simulink library "EmE_MBD_Blockset"  (R2018a)
settings: Solver=ode1  StartTime=0.0  StopTime=Inf  FixedStep=0.001  RelTol=1e-3  EnableMultiTasking=on
PostLoadFcn:
  | , if any(exist('dsrtsu_mdlpostloadfcn', 'file') == [2, 3, 6]), try dsrtsu_mdlpostloadfcn('Execute', bdroot); catch fprintf('Error in PostLoadFcn (dsrtsu_mdlpostloadfcn) for model "%s":\n %s\n', bdroot, lasterr); end, end,
undefined symbols (not defined in the file or in its folder): ENUM_TSC1_CONTROL_PURPOSE_T, gcbh, GLB_SWITCH_T
libraries: simulink x237, $bdroot x115, simulink_need_slupdate x26, MotoHawk_lib x13, simulink_extras x3
(part 1 of 11)
settings Model: DSRTSU_INTERNAL_RTI_VER=520  DSRTSU_INTERNAL_RTI_TYPE=rti1401  DSRTSU_INTERNAL_RTIFPGA=110  RTICANMMDATA=struct('GeneralSetupData',struct('modelroot','C:\data\svn\PowerTrainSys\trunk\src\Projects_RCP\MY2017_RCP\EmE_MBD_Blockset','generalsettings',struct('filesettings',struct('destfolder',struct('Name','RTICANMM_FILES','Check',1),'buildfolder',struct('Name','.','Check',1),'AbsDestfolder',struct('Name','C:\data\svn\PowerTrainSys\trunk\src\Projects_RCP\MY2017_RCP\EmE_MBD_Blockset\RTICANMM_FILES'),'AbsBuildfolder',struct('Name','C:\data\svn\PowerTrainSys\trunk\src\Projects_RCP\MY2017_RCP\EmE_MBD_Blockset'))),'options',struct('addpaths',1,'rmpaths',1,'addtrcexclusion',logical(1),'cannavigator',struct('checkmonitoring',0),'show_usrtrc',0,'use_usrtrc',0),'advanced',struct('options',[1 1 1 1 1 1 1 1 1 1 1 1 1 1 1 1 1 1 1 1 1 1 1 1 1 1 1 1 1 1 1 1 1 1 1 1 1 1 1 1 1 1 1 1 1 1 1 1 1 1 1 1 1 1 1 1 1 1 1 1 1 1 1 1 1 1 1 1 1 1 1 1 1 1 1 1 1 1 1 1 1 1 1 1 1 1 1 1 1 1 1 1 1 1 1 1 1 1 1 1]),'MPSetup',{{}},'modelname','EmE_MBD_Blockset','block','EmE_MBD_Blockset'))  DSRTSU_INTERNAL_RTIFLEXRAYCONFIG=110  Creator=Charles.Swart  LastModifiedBy=Charles.Swart
settings DataIOCC: LimitDataPoints=on  SaveFormat=Array
settings OptimizationCC: BlockReduction=off  OptimizeBlockIOStorage=off  BufferReuse=off  GlobalBufferReuse=off  ExpressionFolding=off  LocalBlockOutputs=off  LifeSpan=inf  OptimizeDataStoreBuffers=off  BusAssignmentInplaceUpdate=off
settings DebuggingCC: SolverPrmCheckMsg=warning  SFUnexpectedBacktrackingDiag=warning  SFNoUnconditionalDefaultTransitionDiag=warning  SFExecutionAtInitializationDiag=none
settings HardwareCC: ProdBitPerPointer=32  ProdBitPerSizeT=32  ProdBitPerPtrDiffT=32  ProdLargestAtomicInteger=Integer  ProdEndianess=BigEndian  ProdWordSize=32  ProdHWDeviceType=Generic->Custom  TargetIntDivRoundTo=Zero  TargetEndianess=BigEndian  TargetHWDeviceType=Generic->Custom
settings ModelReferenceCC: PropagateSignalLabelsOutOfModel=off
settings SFSimCC: MATLABDynamicMemAlloc=off
settings RTWCC: SystemTargetFile=rti1401.tlc  MakeCommand=make_rti  TemplateMakefile=rti1401.tmf  Description=dSPACE DS1401 Hardware Platform
settings CodeAppCC: StateflowObjectComments=on
settings STFCustomTargetCC: ParMdlRefBuildCompliant=on  GeneratePreprocessorConditionals=Disable all  MatFileLogging=on  GRTInterface=off  SystemTargetFile=rti1401.tlc
settings GRTTargetCC: TargetLangStandard=C89/C90 (ANSI)  CompOptLevelCompliant=off  ConcurrentExecutionCompliant=off  GeneratePreprocessorConditionals=Disable all  CombineOutputUpdateFcns=off  CPPClassGenCompliant=off  UseToolchainInfoCompliant=off  ExtModeMexFile=noextcomm
settings ConfigComp: CovMetricSettings=dw  CovHtmlReporting=on  CovSaveCumulativeToWorkspaceVar=on  CovSaveSingleToWorkspaceVar=on  CovExternalEMLEnable=off  CovSFcnEnable=off

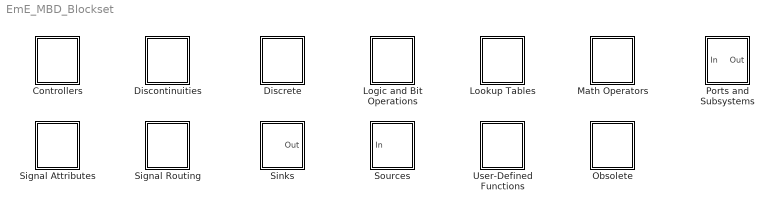
== system EmE_MBD_Blockset ==
  Controllers : Subsystem  mask(Define discontinuous states){}
      mask Display: image(imread('control.bmp','bmp'))
  Discontinuities : Subsystem  mask(Define discontinuous states){}
      mask Display: image(imread('nonlinear.bmp','bmp'))
  Discrete : Subsystem  mask(Define discrete states){}
      mask Display: image(imread('discrete.bmp','bmp'))
  Logic and Bit Operations : Subsystem  mask(Perform logic and bit operations){}
      mask Display: image(imread('logical_bit.bmp','bmp'))
  Lookup Tables : Subsystem  mask(Support lookup tables){}
      mask Display: image(imread('functions.bmp','bmp'))
  Math Operators : Subsystem  mask(Perform math operations){}
      mask Display: image(imread('math.bmp','bmp'))
  Obsolete : Subsystem  mask(Obsolete functions){}
      mask Display:
      | color('gray')
      | disp('X X X')
  Ports and Subsystems : Subsystem  mask(Support ports and subsystems){}
      mask Display: image(imread('subsystems.bmp','bmp'))
  Signal Attributes : Subsystem  mask(Support signal attributes){}
      mask Display: image(imread('attributes.bmp','bmp'))
  Signal Routing : Subsystem  mask(Support signal routing){}
      mask Display: image(imread('signals.bmp','bmp'))
  Sinks : Subsystem  mask(Receive output from other blocks){}
      mask Display: image(imread('sinks.bmp','bmp'))
  Sources : Subsystem  mask(Input to other blocks){}
      mask Display: image(imread('sources.bmp','bmp'))
  User-Defined Functions : Subsystem  mask(User-defined functions){}
      mask Display: image(imread('functions.bmp','bmp'))

== system EmE_MBD_Blockset/Controllers ==
  Generic_PID_Governor_3 : Subsystem  mask(Generic PID governor v3){}
      mask help:
      | Generic feedback governor v3 with proportional, integral, and derivative action (PID).
      | Anti-windup is achieved with a specified hysteresis limit value and a toggleable output unlimited vs. output limited delta feedback.
      | Derivative action has a optional configurable parameter to operate at specified multiples of the dT.
      | If GPID_slew_init is connected to GPID_setpoint, then the GPID_control_error value will be =(GPID_setpoint-GPID_feedback) upon a reset.
      | If GPID_slew_init is connected to GPID_feedback, then the GPID_control_error value will be =0 upon a reset.
      |
      | Do NOT connect GPID_slew_init to the GPID_setpoint port if using negative gains; else the integrator will initialize with a large negative value.
  Generic_PID_Governor_4 : Subsystem  mask(Generic PID governor 4 (EmE)){}
      mask help:
      | Generic feedback governor v4 with proportional, integral, and derivative action (PID).
      | Anti-windup is achieved with a specified hysteresis limit value and a toggleable output unlimited vs. output limited delta feedback.
      | Derivative action has a optional configurable parameter to operate at specified multiples of the dT.
      | If GPID_slew_init is connected to GPID_setpoint, then the GPID_control_error value will be =(GPID_setpoint-GPID_feedback) upon a reset.
      | If GPID_slew_init is connected to GPID_feedback, then the GPID_control_error value will be =0 upon a reset.
      |
      | Do NOT connect GPID_slew_init to the GPID_setpoint port if using negative gains; else the integrator will initialize with a large negative value.
      mask Display: % GPID_AW_USE_FEEDBACK_DELTA_CPV
  PID_saturating_terms : Subsystem  mask(PID governor (EmE)){}
      mask help:
      | PID governor with proportional, integral, and derivative action (PID).
      | Anti-windup is achieved with saturating P, I, and D terms.

== system EmE_MBD_Blockset/Discontinuities ==
  Debounce : Subsystem  mask(Debounce (EmE)){}
      mask help:
      | Performs a signal debounce using ON_T and OFF_T threshold values in seconds.
      | If IN == TRUE for at least ON_T seconds AND OUT(prev) = FALSE, then OUT = TRUE.
      | If IN == FALSE for at least OFF_T seconds AND OUT(prev) = TRUE, then OUT = FALSE
      mask Display:
      | % input bouncy
      | plot([0.25 0.30 0.30],[0.55 0.55 0.75])
      | plot([0.30 0.32 0.32],[0.75 0.75 0.55])
      | plot([0.32 0.34 0.34],[0.55 0.55 0.75])
      | plot([0.34 0.36 0.36],[0.75 0.75 0.55])
      | plot([0.36 0.38 0.38],[0.55 0.55 0.75])
      | plot([0.38 0.55 0.55],[0.75 0.75 0.55])
      | 
      | 
      | plot([0.56 0.58 0.58 0.60],[0.55 0.55 0.75 0.75])
      | 
      | 
      | plot([0.61 0.62 0.62],[0.55 0.55 0.75])
      | plot([0.61 0.61],[0.75 0.55])
      | plot([0.62 0.64 0.64 0.80],[0.75 0.75 0.55 0.55])
      | 
      | % output
      | plot([0.25 0.40 0.40],[0.25 0.25 0.45])
      | plot([0.40 0.68 0.68 0.80],[0.45 0.45 0.25 0.25])
  Dynamic_saturation : Subsystem  mask(Dynamic saturation (EmE)){}
      mask help: Bound the range of the second input by using the first input (upper limit) and the third input (lower limit).
      mask Display: plot([0.2 0.8],[.5 .5],[.5 .5],[0.05 0.95],0.15+0.7*[0 .25 .75 1],0.05+0.9*[.25 .25 .75 .75]);
  Falling_edge : Subsystem  mask(Falling edge (EmE)){initact=off}
      mask prompts: initact "Act on initial condition (= false)"
      mask help:
      | Detects a falling edge on a logical signal giving output TRUE for one sample.
      | In: FALSE -> TRUE      Out: FALSE
      | In: TRUE  -> FALSE     Out: TRUE
      | In: FALSE -> FALSE     Out: FALSE
      | In: TRUE  -> TRUE      Out: FALSE
      mask init:
      | unitdelay = [get_param(gcbh,'parent'),'/',get_param(gcbh,'name'),'/Unit_Delay'];
      | if strcmp(initact,'on')
      |     set_param(unitdelay,'InitialCondition','true');
      | else
      |     set_param(unitdelay,'InitialCondition','false');
      | end
      settings: AttributesFormatString=Action on IC: %<initact>
      mask Display:
      | plot([0.1 0.5],[0.9 0.9])
      | plot([0.5 0.5],[0.1 0.9])
      | plot([0.5 0.9],[0.1 0.1])
      | plot([0.4 0.5 0.6],[0.6 0.4 0.6])
  Hysteresis : Subsystem  mask(Hysteresis (EmE)){hyst_init=false, init_val=false}
      mask prompts: hyst_init "Initial value:"; init_val "dummy value:"
      mask help:
      | The output is set to TRUE when the input reaches the 'High' threshold and is set to FALSE when the input drops below the 'Low' threshold.
      | In                            Previous_Out        Out
      | In >= High                     n/a               TRUE
      | Low < In < High          TRUE              TRUE
      | Low < In < High          FALSE             FALSE
      | In <= Low                      n/a              FALSE
      mask init:
      | if strcmp(hyst_init,'false')
      |     init_val = 'false';
      |     set_param(gcbh,'init_val',init_val);
      | elseif strcmp(hyst_init,'true')
      |     init_val = 'true';
      |     set_param(gcbh,'init_val',init_val);
      | end
      | unit_delay = [get_param(gcbh,'parent'),'/',get_param(gcbh,'name'),'/Unit_Delay'];
      | set_param(unit_delay,'InitialCondition',init_val);
      mask TypeOptions hyst_init: true | false
      mask Display:
      | plot([0.2 0.6],[0.1 0.1])
      | plot([0.6 0.6],[0.1 0.9])
      | plot([0.4 0.8],[0.9 0.9])
      | plot([0.55 0.6 0.65],[0.45 0.55 0.45])
      | 
      | plot([0.4 0.4],[0.1 0.9])
      | plot([0.35 0.4 0.45],[0.55 0.45 0.55])
  Rising_edge : Subsystem  mask(Rising edge (EmE)){initact=off}
      mask prompts: initact "Act on initial condition (= true)"
      mask help:
      | Detects a rising edge on a logical signal giving output TRUE for one sample.
      | In: FALSE -> TRUE      Out: TRUE
      | In: TRUE  -> FALSE     Out: FALSE
      | In: FALSE -> FALSE     Out: FALSE
      | In: TRUE  -> TRUE      Out: FALSE
      mask init:
      | unitdelay = [get_param(gcbh,'parent'),'/',get_param(gcbh,'name'),'/Unit_Delay'];
      | if strcmp(initact,'on')
      |     set_param(unitdelay,'InitialCondition','false');
      | else
      |     set_param(unitdelay,'InitialCondition','true');
      | end
      settings: AttributesFormatString=Action on IC: %<initact>
      mask Display:
      | plot([0.1 0.5],[0.1 0.1])
      | plot([0.5 0.5],[0.1 0.9])
      | plot([0.5 0.9],[0.9 0.9])
      | plot([0.4 0.5 0.6],[0.4 0.6 0.4])

== system EmE_MBD_Blockset/Discrete ==
  DT1_Derivative_lag : Subsystem  mask(DT1 filter (EmE)){}
      mask help: This element has a step response which initially contains a step and then decreases exponential to zero with a characteristic time constant.
      mask Display:
      | plot([0.2 0.2], [0.2 0.8]); % y axis
      | plot([0.2 0.9], [0.2 0.2]); % x axis
      | plot([0.2 0.22], [0.2 0.7]);
      | plot([0.22 0.27], [0.7 0.45]);
      | plot([0.27 0.33], [0.45 0.29]);
      | plot([0.33 0.37], [0.29 0.25]);
      | plot([0.37 0.4], [0.25 0.23]);
      | plot([0.4 0.5], [0.23 0.21]);
      | plot([0.5 0.65],[0.21 0.21]);
      | plot([0.65 0.9],[0.21 0.21]);
  Discrete Derivative : Subsystem  mask(Discrete derivative (EmE)){}
      mask help:
      | Discrete-time derivative of the input.
      | u is the input.
      | IC is the initial condition input.
      | K is the gain value.
      | dT is the sample time in seconds.
      | y is the output.
      |
      |
      | At the first time step, the calculation is as follows:
      | y(1) = [(K*u(1))/dT] - u(0)
      |
      | Otherwise, the calculation is as follows:
      | y(n) = [(K*u(n))/dT] - [(K*u(n-1))/dT]
      |
      | where:
      | u(n)=input at current time step
      | u(n-1)=input at previous time step
      | u(0)=value at initial condition input (used for first time step only)
      | y(n)=output at current time step
      | K=scaling factor
      | dT=sample time in seconds
      mask Display:
      | text(0.5, 0.5, 'K(z-1)', 'horizontalAlignment', 'center', 'verticalAlignment', 'bottom');
      | text(0.5, 0.5, 'Ts z', 'horizontalAlignment', 'center', 'verticalAlignment', 'top')
      | plot([0.3 0.7],[0.5 0.5]);
      | port_label('input',1,'u');
      | port_label('input',2,'IC');
      | port_label('input',3,'K');
      | port_label('input',4,'dT');
      | port_label('output',1,'y');
  Discrete-Time Integrator : Subsystem  mask(Discrete-time integrator (EmE)){integrator_method_sel=Backward Euler}
      mask prompts: integrator_method_sel "Integrator method:"
      mask help:
      | Discrete-time integration or accumulation of the input signal.
      | F_Reset is the reset Boolean input.
      | u is the input.
      | K is the gain value.
      | dT is the sample time in seconds.
      | y is the output.
      |
      | A reset condition causes the accumlated output to be reset to zero.
      |
      |
      | The calculation is as follows:
      | Forward Euler: y(n) = y(n-1) + K*dT*u(n-1)
      | Backward Euler: y(n) = y(n-1) + K*dT*u(n)
      | Trapezoidal: y(n) = y(n-1) + K*dT*[u(n)+u(n-1)]/2
      |
      | where:
      | u(n)=input at current time step
      | u(n-1)=input at previous time step
      | y(n)=output at current time step
      | y(n-1)=output at previous time step
      | K=scaling factor
      | dT=sample time in seconds
      mask init:
      | % assign values in simulink block
      | % reset_method = [get_param(gcbh,'Parent'),'/',get_param(gcbh,'name'),'/Reset_method/Reset_method'];
      | integrator_method = [get_param(gcbh,'Parent'),'/',get_param(gcbh,'name'),'/Integrator_method/Integrator_method'];
      | % integration_method = [get_param(gcbh,'Parent'),'/',get_param(gcbh,'name'),'/Integration_or_accumulation/Integration_method'];
      | 
      | % assign numbers to selected values
      | % switch reset_method_sel
      | %     case 'rising edge', reset_method_value = 1; % 'rising edge'
      | %     case 'falling edge', reset_method_value = 2; % 'falling edge'
      | %     case 'either edge', reset_method_value = 3; % 'either edge'
      | %     case 'level', reset_method_value = 4; % 'level'
      | % end;
      | switch integrator_method_sel
      |     case 'Forward Euler', integrator_method_value = 2; % 'Forward Euler'
      |     case 'Backward Euler', integrator_method_value = 1; % 'Backward Euler'
      |     case 'Trapezoidal', integrator_method_value = 3; % 'Trapezoidal'
      | end;
      | % switch integration_method_sel
      | %     case 'Integration (use external dT)', integration_method_value = true; % 'Integration (use external dT)'
      | %     case 'Accumulation (dT=1)', integration_method_value = false; % 'Accumulation (dT=1)'
      | % end;
      | 
      | % set params
      | % set_param(reset_method, 'Value', num2str(reset_method_value));
      | set_param(integrator_method, 'Value', num2str(integrator_method_value));
      | % set_param(integration_method, 'Value', num2str(integration_method_value));
      settings: AttributesFormatString=%<integrator_method_sel>
      mask TypeOptions integrator_method_sel: Forward Euler | Backward Euler | Trapezoidal
      mask Display:
      | text(0.5, 0.5, 'K Ts', 'horizontalAlignment', 'center', 'verticalAlignment', 'bottom');text(0.5, 0.5, 'z-1', 'horizontalAlignment', 'center', 'verticalAlignment', 'top');plot([0.3 0.7],[0.5 0.5]);
      | port_label('input',1,'F_Reset');
      | port_label('input',2,'u');
      | % port_label('input',3,'IC_u');
      | % port_label('input',4,'IC_y');
      | port_label('input',3,'K');
      | port_label('input',4,'dT');
      | port_label('output',1,'y');
  Exponential_weighted_average : Subsystem  mask(Exponentially weighted average (EmE)){}
      mask help:
      | Computes a set of weights and applies these weights to the data samples recursively.
      | As the age of the data increases, the magnitude of the weighting factor decreases exponentially and never reaches zero.
      | In other words, the recent data has more influence on the statistic at the current sample than the older data.
      | Due to the infinite impulse response, the algorithm requires fewer coefficients, making it more suitable for embedded applications.
      | K = Forgetting factor (must be: 0.001<K<1)
  Frequency_detector : Subsystem  mask(Frequency detector (EmE)){}
      mask help:
      | Outputs an input signal's frequency in Hz.
      | If F_Trigger_Select is TRUE, then triggers on rising edge if Signal_In is above or equal to Trigger_Level.
      | If F_Trigger_Select is FALSE, then triggers on falling edge if Signal_In is below or equal to Trigger_Level.
      | If Signal_In does not cause a trigger within Timeout_T seconds, then Out_Freq_Hz will be 0.
      | dT is the dynamic sample rate in seconds.
  LPF_first_order : Subsystem  mask(Low pass filter, first order (EmE)){}
      mask help:
      | Discrete first order low-pass filter with time constant T [sec].
      | Filters the input to smooth out high frequent or random noise.
      | Can be reset to a custom initial value (Init).
      mask Display:
      | plot([0.4  0.4], [0.2 0.8]);
      | plot([0.4 0.9], [0.2 0.2]);
      | plot([0.4 0.6], [0.7 0.7]);
      | plot([0.6  0.8], [0.7 0.2]);
      | plot([0.6 0.6],[0.65 0.6]);
      | plot([0.6 0.6],[0.55 0.5]);
      | plot([0.6 0.6],[0.45 0.4]);
      | plot([0.6 0.6],[0.35 0.3]);
      | plot([0.6 0.6],[0.25 0.2]);
      | text(0.25,0.69,'0 dB')
      | text(0.58,0.15,'f')
      | text(0.60,0.13,'c')
  One_shot_pulse : Subsystem  mask(One-shot pulse (EmE)){}
      mask help:
      | Triggers a one-shot pulse of fixed duration when the input is TRUE.
      |
      | Duration: duration of the pulse (seconds)
      | dT: dynamic sample rate (seconds)
      mask Help:
      | If the duration input is less than the dT input, the output will be FALSE.
      | Else: on the rising edge of the In input, a single-shot output will be made with a length (in seconds) specified at the Duration input.
      mask Display:
      | plot([0.2 0.3 0.3 0.4 0.4 0.8],[0.7 0.7 0.9 0.9 0.7 0.7])
      | plot([0.2 0.3 0.3 0.7 0.7 0.8],[0.2 0.2 0.4 0.4 0.2 0.2])
      | 
      | plot([0.3 0.7],[0.3 0.3])
      | plot([0.35 0.3 0.35],[0.25 0.3 0.35])
      | plot([0.65 0.7 0.65],[0.25 0.3 0.35])
      | 
      | text(0.37, 0.15, 'duration')
  PT1_First_order_lag : Subsystem  mask(PT1 filter (EmE)){}
      mask help: The 1st-order lag element outputs a signal that, for a step input, has a certain initial slope and approaches asymptotically the final value.
      mask Display:
      | plot([0.2 0.2], [0.2 0.8]); % y axis
      | plot([0.2 0.9], [0.2 0.2]); % x axis
      | plot([0.2 0.3], [0.2 0.5]);
      | plot([0.3 0.35], [0.5 0.6]);
      | plot([0.35 0.4], [0.6 0.65]);
      | plot([0.4 0.5], [0.65 0.7]);
      | plot([0.5 0.65],[0.7 0.72]);
      | plot([0.65 0.9],[0.72 0.72]);
  Savitzky-Golay_Diff_Filter : Subsystem  mask(Savitzky Golay Diff Filter (EmE)){}
      mask help: The Savitzky–Golay smoothing filter is a filter that essentially performs a local polynomial regression on a series of values to determine the smoothed value for each point.
  Sliding_window_average : Subsystem  mask(Sliding window average (EmE)){kfactor=4}
      mask prompts: kfactor "Window length:"
      mask help:
      | A window of specified length moves over the data, sample by sample, and the statistic is computed over the data in the window.
      | The output for each input sample is the statistic over the window of the current sample and the window length -1 previous samples.
      | In the first-time step, to compute the first window length -1 outputs when the window does not have enough data yet, the algorithm fills the window with zeros.
      | In the subsequent time steps, to fill the window, the algorithm uses samples from the previous data frame.
      | The moving statistic algorithms have a state and remember the previous data.
      mask init:
      | constant = [get_param(gcbh,'parent'),'/',get_param(gcbh,'name'),'/Constant'];
      | set_param(constant,'Value',['ones(1,' floor(kfactor) ')']);
      settings: AttributesFormatString=Window length: %<kfactor>
  Timer_enabled_with_reset : Subsystem  mask(Timer enabled with reset (EmE)){}
      mask help: A timer block that outputs elapsed time and time remaining.
      mask init:
      | alpha=0:2*pi/100:2*pi;
      mask Display:
      | plot(0.5+0.3*cos(alpha),0.5+0.3*sin(alpha));
      | plot(0.5+[0.3*cos(pi/2),0,0.3*cos(-pi/4)],0.5+[0.3*sin(pi/2),0,0.3*sin(-pi/4)]);
      | plot([0.5-0.1*0.707 0.5 0.5+0.1*0.707],[0.7 0.8 0.7])
      | plot([0.62 0.71 0.71],[0.29 0.29 0.38])
  Turn_off_delay : Subsystem  mask(Turn-off delay (EmE)){}
      mask help:
      | Delays the falling edge of the input signal by a specified duration; rising edge is synchronized with the input.
      |
      | Duration: duration to delay output to off (seconds)
      | dT: dynamic sample rate (seconds)
      mask Display:
      | plot([0.2 0.3 0.3 0.75 0.75 0.8],[0.9 0.9 0.7 0.7 0.9 0.9])
      | plot([0.2 0.5 0.5 0.75 0.75 0.8],[0.4 0.4 0.2 0.2 0.4 0.4])
      | 
      | plot([0.3 0.5],[0.3 0.3])
      | plot([0.35 0.3 0.35],[0.25 0.3 0.35])
      | plot([0.45 0.5 0.45],[0.25 0.3 0.35])
      | 
      | text(0.27, 0.18, 'duration')
  Turn_on_delay : Subsystem  mask(Turn-on delay (EmE)){}
      mask help:
      | Delays the rising edge of the input signal by a specified duration; falling edge is synchronized with the input.
      |
      | Duration: duration to delay output to on (seconds)
      | dT: dynamic sample rate (seconds)
      mask Display:
      | plot([0.2 0.3 0.3 0.75 0.75 0.8],[0.7 0.7 0.9 0.9 0.7 0.7])
      | plot([0.2 0.5 0.5 0.75 0.75 0.8],[0.2 0.2 0.4 0.4 0.2 0.2])
      | 
      | plot([0.3 0.5],[0.3 0.3])
      | plot([0.35 0.3 0.35],[0.25 0.3 0.35])
      | plot([0.45 0.5 0.45],[0.25 0.3 0.35])
      | 
      | text(0.2, 0.4, 'duration')
  Unit Delay Enabled : simulink_need_slupdate/Unit Delay Enabled  vinit=false  tsamp=-1
      settings: AttributesFormatString=IC: %<vinit>  SourceProductName=Simulink  SourceProductBaseCode=SL
  Unit Delay Enabled External IC : simulink_need_slupdate/Unit Delay Enabled External IC  tsamp=-1
      settings: SourceProductName=Simulink  SourceProductBaseCode=SL
  Unit Delay Enabled Resettable : simulink_need_slupdate/Unit Delay Enabled Resettable  vinit=false  tsamp=-1
      settings: AttributesFormatString=IC: %<vinit>  SourceProductName=Simulink  SourceProductBaseCode=SL
  Unit Delay Enabled Resettable External IC : simulink_need_slupdate/Unit Delay Enabled Resettable External IC  tsamp=-1
      settings: SourceProductName=Simulink  SourceProductBaseCode=SL
  Unit Delay External IC : simulink_need_slupdate/Unit Delay External IC  tsamp=-1
      settings: SourceProductName=Simulink  SourceProductBaseCode=SL
  Unit Delay Resettable : simulink_need_slupdate/Unit Delay Resettable  vinit=false  tsamp=-1
      settings: AttributesFormatString=IC: %<vinit>  SourceProductName=Simulink  SourceProductBaseCode=SL
  Unit Delay Resettable External IC : simulink_need_slupdate/Unit Delay Resettable External IC  tsamp=-1
      settings: SourceProductName=Simulink  SourceProductBaseCode=SL
  Unit_Delay : UnitDelay  InitialCondition=false  SampleTime=-1
      settings: AttributesFormatString=IC: %<vinit>

== system EmE_MBD_Blockset/Logic and Bit Operations ==
  Bitwise Operator : simulink/Logic and Bit Operations/Bitwise Operator  logicop=AND  UseBitMask=on  BitMask=bin2dec('11011001')  BitMaskRealWorld=Stored Integer
  Compare To Constant : simulink/Logic and Bit Operations/Compare To Constant  relop=<=  const=3  OutDataTypeStr=boolean
  Compare To Constant1 : simulink/Logic and Bit Operations/Compare To Constant  relop===  const=ENUM_TSC1_CONTROL_PURPOSE_T.P1_ACCELERATOR_OPERATOR  OutDataTypeStr=boolean
  Compare To Zero : simulink/Logic and Bit Operations/Compare To Zero  relop=<=  OutDataTypeStr=boolean
  D flip-flop : simulink_extras/Flip Flops/D Flip-Flop
      settings: SourceProductName=Simulink
  D flip-flop with SR : Subsystem  mask(D flip-flop with SR (EmE)){}
      mask help:
      | D flip-flop with set-reset override.
      | If S OR R input is TRUE, then CLK, D, and !CLR inputs are ignored and outputs are overridden per truth table.
      | If S AND R are FALSE, then block works as a typical D flip-flop.
      mask Help:
      | Legend:
      | R=Rising edge
      | N=Non-rising edge
      | X=Don't care
      | 
      | Truth table:<font face="courier">
      | CLK D   !CLR S   R   Q   !Q
      | R   0   1    0   0   0   1
      | R   1   1    0   0   1   0
      | N   X   1    0   0   Q   !Q
      | X   X   0    0   0   0   1
      | X   X   X    0   1   0   1
      | X   X   X    1   0   1   0
      | X   X   X    1   1   1   1
      | </font>
  Detect Change : simulink/Logic and Bit Operations/Detect Change  vinit=0  InputProcessing=Inherited  OutDataTypeStr=boolean
      settings: AttributesFormatString=IC: %<vinit>
  Detect Decrease : simulink/Logic and Bit Operations/Detect Decrease  vinit=0  InputProcessing=Inherited  OutDataTypeStr=boolean
      settings: AttributesFormatString=IC: %<vinit>
  Detect Increase : simulink/Logic and Bit Operations/Detect Increase  vinit=0  InputProcessing=Inherited  OutDataTypeStr=boolean
      settings: AttributesFormatString=IC: %<vinit>
  Gated D latch : simulink_extras/Flip Flops/D Latch
      settings: SourceProductName=Simulink  SourceProductBaseCode=SL
  JK flip-flop : simulink_extras/Flip Flops/J-K Flip-Flop  initial_condition=false
      settings: AttributesFormatString=IC: %<initial_condition>  SourceProductName=Simulink
  Logical Operator : Logic  Inputs=Inputs  OutDataTypeStr=boolean  mask(Logical operator (EmE)){Operator=AND, Inputs=2}
      mask prompts: Operator "Simulink:blkprm_prompts:LogicOperator"; Inputs "Simulink:blkprm_prompts:LogicNumInputPorts"
      mask help: Logical operators. For a single input, operators are applied across the input vector. For multiple inputs, operators are applied across the inputs.
      mask TypeOptions Operator: Operator
      mask TypeOptions Inputs: Inputs
      mask DialogControl Operator Prompt: Operator:
      mask DialogControl Inputs Prompt: Number of input ports:
  RS flip-flop : Subsystem  mask(RS flip-flop (EmE)){}
      mask help: RS flip-flop with priority on reset input.
      mask Help:
      | Truth table:<font face="courier">
      | S R Q !Q
      | 0 0 Q !Q
      | 0 1 0  1
      | 1 0 1  0
      | 1 1 0  1
      | </font>
  Relational Operator : RelationalOperator  Operator===  OutDataTypeStr=boolean  RndMeth=Nearest  InputSameDT=on  mask(Relational operator (EmE)){func===}
      mask prompts: func "Relational operator:"
      mask help: Applies the selected relational operator to the inputs and outputs the result. The top (or left) input corresponds to the first operand.
      mask init:
      | set_param(gcb,'operator',func)
      mask TypeOptions func: == | ~= | < | <= | >= | >
  SR flip-flop : Subsystem  mask(SR flip-flop (EmE)){}
      mask help: SR flip-flop with priority on set input.
      mask Help:
      | Truth table:<font face="courier">
      | S R Q !Q
      | 0 0 Q !Q
      | 0 1 0  1
      | 1 0 1  0
      | 1 1 1  0
      | </font>
  Shift Arithmetic : ArithShift  BitShiftNumber=8

== system EmE_MBD_Blockset/Lookup Tables ==
  1-D Lookup Table : Lookup_n-D  NumberOfTableDimensions=1  BreakpointsForDimension1=[1 2 3]  Table=[1 9 6]  ExtrapMethod=Clip  UseLastTableValue=on  InputSameDT=on  mask(Lookup table X1D (EmE)){maskInput=[1 2 3], maskTableData=[1 9 6]}
      mask prompts: maskInput "Vector of input values (X) (input):"; maskTableData "Table data (Y) (output):"
      mask help:
      | Perform 1-D linear interpolation of input values using the specified table.
      | Extrapolation is forbidden and end-values are used when exceeding the 'Table data' boundaries.
      mask init:
      | set(gcbh,'BreakpointsForDimension1', maskInput,'Table', maskTableData)
      settings: AttributesFormatString=|
      | X: %<BreakpointsForDimension1>
      | Y: %<Table>
  2-D Lookup Table : Lookup_n-D  BreakpointsForDimension1=[1 2 3]  BreakpointsForDimension2=[2 4 6]  ExtrapMethod=Clip  UseLastTableValue=on  InputSameDT=on  mask(Lookup table X2D (EmE)){maskRowValues=[1 2 3], maskColValues=[2 4 6], maskTableData=[4 5 6;16 19 20;10 18 23]}
      mask prompts: maskRowValues "Vector of column input (X) values (input u1):"; maskColValues "Vector of row input (Y) values (input u2):"; maskTableData "Table data (Z) (output):"
      mask help:
      | Performs 2-D linear interpolation of input values using the specified table.
      | X values (columns) correspond to the upper input port, u1.
      | Y values (rows) correspond to the lower input port, u2.
      | Extrapolation is forbidden and end-values are used when exceeding the 'Table data' boundaries.
      mask init:
      | set(gcbh,'BreakpointsForDimension1', maskRowValues, 'BreakpointsForDimension2', maskColValues, 'Table', maskTableData)
      settings: AttributesFormatString=|
      | X: %<BreakpointsForDimension1>
      | Y: %<BreakpointsForDimension2>
      | Z: %<Table>
